simulink model "mbed_analogInOut"  (R2015a)
settings: Solver=FixedStepDiscrete  SolverMode=SingleTasking  StartTime=0.0  StopTime=10.0  FixedStep=1e-3  RelTol=1e-3
libraries: mbed_lib x5, mbed_targets_stm_disco_f407 x3, simulink x1
settings Model: CovSFcnEnable=off  Creator=oh  LastModifiedBy=oh
settings OptimizationCC: OptimizeModelRefInitCode=on  LifeSpan=1
settings DebuggingCC: SolverPrmCheckMsg=warning
settings HardwareCC: ProdLargestAtomicInteger=Long  ProdLargestAtomicFloat=Double  ProdEndianess=LittleEndian  ProdHWDeviceType=ARM Compatible->ARM Cortex
settings RTWCC: SystemTargetFile=mbed.tlc  TemplateMakefile=mbed.tmf  Description=Mbed Target (Embedded Target)  TargetLang=C++
settings CodeAppCC: IgnoreCustomStorageClasses=off
settings STFCustomTargetCC: CombineOutputUpdateFcns=on  SupportVariableSizeSignals=off  SystemTargetFile=mbed.tlc
settings ERTTargetCC: SupportVariableSizeSignals=off  ERTCustomFileTemplate=mbed_file_process.tlc

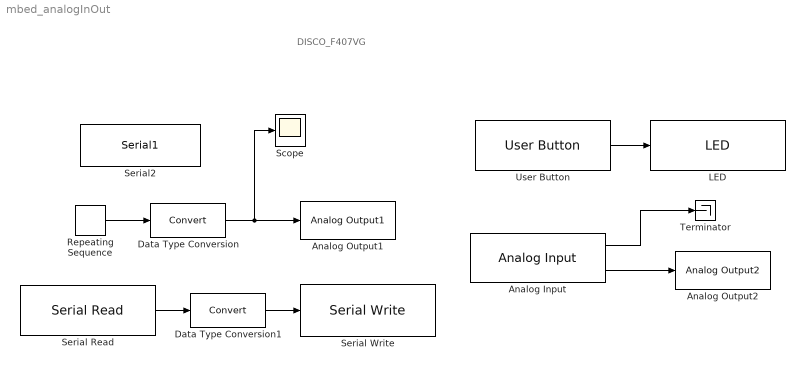
== system mbed_analogInOut ==
  note: DISCO_F407VG
  Analog Input : mbed_lib/GPIO/Analog Input  PortName=A  PinNumber=0  SampleTime=0.1
  Analog Output1 : mbed_targets_stm_disco_f407/Analog Output1  Parameter1=0
  Analog Output2 : mbed_targets_stm_disco_f407/Analog Output2
  Data Type Conversion : DataTypeConversion
  Data Type Conversion1 : DataTypeConversion
  LED : mbed_lib/GPIO/LED  nLED=1  SampleTime=-1
  Repeating Sequence : simulink/Sources/Repeating Sequence  rep_seq_t=[0 2]  rep_seq_y=[0 1]
  Scope : Scope
  Serial Read : mbed_lib/Serial/Serial Read  SParameter1=1  SampleTime=0.1
  Serial Write : mbed_lib/Serial/Serial Write  SerialPort=1  numData=off  SampleTime=-1
  Serial2 : mbed_targets_stm_disco_f407/Serial1  Parameter1=0  BaudRate=9600
  Terminator : Terminator
  User Button : mbed_lib/GPIO/User Button  SampleTime=0.1
  wires:
  Repeating Sequence/1 -> Data Type Conversion/1
  Analog Input/2 -> Analog Output2/1
  Data Type Conversion/1 -> Analog Output1/1, Scope/1
  Analog Input/1 -> Terminator/1
  User Button/1 -> LED/1
  Data Type Conversion1/1 -> Serial Write/1
  Serial Read/1 -> Data Type Conversion1/1
